simulink model "Steadystate_pmsm"  (R2020a)
settings: Solver=ode4  StartTime=0.0  StopTime=2  FixedStep=1e-4  RelTol=1e-3
PreLoadFcn:
  | % motor parameters
  | rs = 0.2;               %Stator resistance
  | Lq = 300e-6;            %d and q axis inductances
  | Ld = 300e-6;
  | Lambda_m_r = 0.01;      %rotor flux linkages (back-emf constant)
  | P=2;                    % numer of poles
  | % current controller gains
  | BW = 2*pi*(100*0.1592*0.7071); %controller bandwidth in radps
  | Kp = BW*Lq;
  | Ki = BW*rs;
settings Model: Creator=samee
settings DebuggingCC: UnconnectedInputMsg=none  UnconnectedOutputMsg=none  UnconnectedLineMsg=none

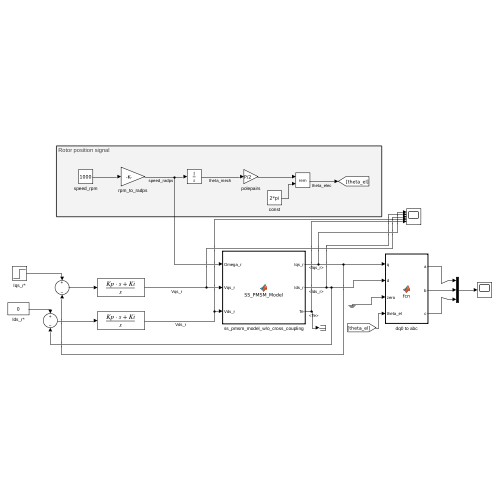
[thumbnail: Simulink's stored preview of the top-level diagram]
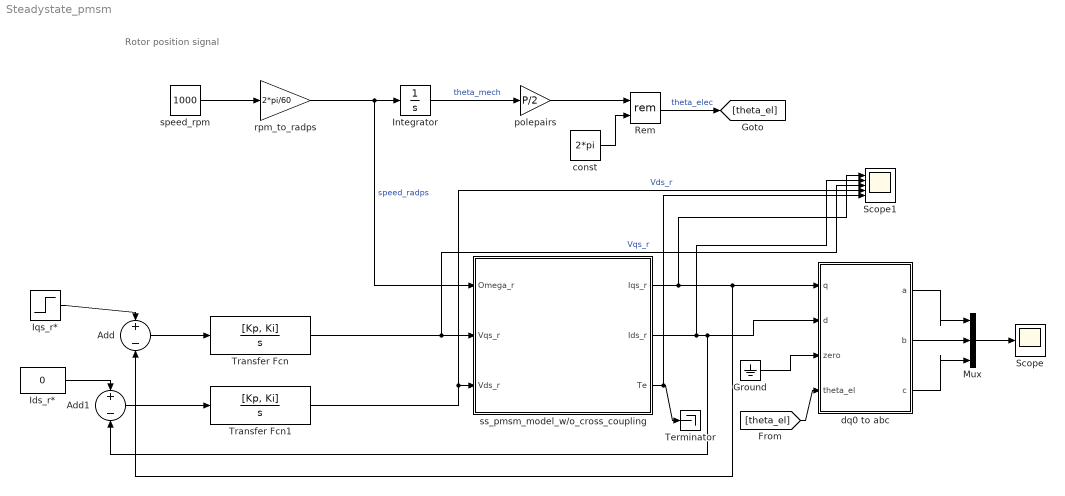
== system Steadystate_pmsm ==
  note: Rotor position signal
  Add : Sum  Inputs=+-
  Add1 : Sum  Inputs=+-
  Ground : Ground
  Ids_r* : Constant  Value=0
  Integrator : Integrator
  Iqs_r* : Step  After=2  SampleTime=0
  Mux : Mux  Inputs=3
  Rem : Math  Operator=rem  SaturateOnIntegerOverflow=on
  Scope : Scope
  Scope1 : Scope  NumInputPorts=5
  Terminator : Terminator
  Transfer Fcn : TransferFcn  Numerator=[Kp, Ki]  Denominator=[1 0]
  Transfer Fcn1 : TransferFcn  Numerator=[Kp, Ki]  Denominator=[1 0]
  const : Constant  Value=2*pi
  dq0 to abc : MATLAB Function  TreatAsAtomicUnit=on
  polepairs : Gain  Gain=P/2
  rpm_to_radps : Gain  Gain=2*pi/60
  speed_rpm : Constant  Value=1000
  ss_pmsm_model_w/o_cross_coupling : MATLAB Function  TreatAsAtomicUnit=on
  wires:
  Integrator/1 -> polepairs/1  "theta_mech"
  const/1 -> Rem/2
  polepairs/1 -> Rem/1
  speed_rpm/1 -> rpm_to_radps/1
  rpm_to_radps/1 -> Integrator/1, ss_pmsm_model_w/o_cross_coupling/1(Omega_r)  "speed_radps"
  Rem/1 -> [theta_el]  "theta_elec"
  Transfer Fcn/1 -> Scope1/3, ss_pmsm_model_w/o_cross_coupling/2(Vqs_r)  "Vqs_r"
  Transfer Fcn1/1 -> Scope1/4, ss_pmsm_model_w/o_cross_coupling/3(Vds_r)  "Vds_r"
  ss_pmsm_model_w/o_cross_coupling/1(Iqs_r) -> Scope1/1, dq0 to abc/1(q), Add/2
  ss_pmsm_model_w/o_cross_coupling/2(Ids_r) -> Scope1/2, dq0 to abc/2(d), Add1/2
  ss_pmsm_model_w/o_cross_coupling/3(Te) -> Scope1/5, Terminator/1
  Ground/1 -> dq0 to abc/3(zero)
  [theta_el] -> dq0 to abc/4(theta_el)
  Iqs_r*/1 -> Add/1
  Add/1 -> Transfer Fcn/1
  Ids_r*/1 -> Add1/1
  Add1/1 -> Transfer Fcn1/1
  dq0 to abc/2(b) -> Mux/2
  dq0 to abc/1(a) -> Mux/1
  dq0 to abc/3(c) -> Mux/3
  Mux/1 -> Scope/1

== matlab function Steadystate_pmsm/dq0 to abc ==
  data: q input; d input; a output; zero input; theta_el input; b output; c output
function [a, b, c] = fcn(q, d, zero, theta_el)

a = cos(theta_el)*q + sin(theta_el)*d + zero*1;
b = cos(theta_el-(2*pi/3))*q + sin(theta_el-(2*pi/3))*d + zero*1;
c = cos(theta_el+(2*pi/3))*q + sin(theta_el+(2*pi/3))*d + zero*1;

== matlab function Steadystate_pmsm/ss_pmsm_model_w//o_cross_coupling ==
  data: Omega_r input; Vqs_r input; Iqs_r output; Vds_r input; Ids_r output; Te output
function [Iqs_r, Ids_r, Te] = SS_PMSM_Model(Omega_r, Vqs_r, Vds_r)
%#codegen

rs = 0.2;               %Stator resistance
Lq = 300e-6;            %d and q axis inductances
Ld = 300e-6;
Lambda_m_r = 0.01;      %rotor flux linkages (back-emf constant)
P=2;                    % numer of poles   


K1 = ((rs^2) + (Omega_r^2)*Ld*Lq);

% Motor currents in rotor reference frame
Iqs_r = (rs/K1) * (Vqs_r - Omega_r*Lambda_m_r - (Omega_r*Ld/rs)*Vds_r);
Ids_r = (1/K1) * (rs*Vds_r + Omega_r*Lq*Vqs_r - (Omega_r^2)*Lq*Lambda_m_r);

% Electromagnetic torque generated
Te = (3/2)*(P/2)*((Lambda_m_r*Iqs_r) + ((Ld - Lq)*Iqs_r*Ids_r));
